simulink model "app_Main50msMgr"  (R2016b)
settings: Solver=FixedStepDiscrete  StartTime=0.0  StopTime=10.0  FixedStep=0.001  RelTol=1e-3  EnableMultiTasking=on
PreLoadFcn:
  | try
  |    tapas_types('load');
  | catch
  |   disp('TAPAS WARNING: Tapas Types could not be loaded ...');
  | end
  | 
  | try
  |   app_types('load');
  | catch
  |   currdir =pwd;
  |   try
  |     cd('..\app_types\');
  |     app_types('load');
  |     cd(currdir);
  |   catch
  |     try
  |        cd('..\..\app_types\');
  |        app_types('load');
  |        cd(currdir);
  |     catch
  |        cd(currdir);
  |        disp('TAPAS WARNING: Application Types could not be loaded ...');
  |     end
  |   end
  |   try
  |       clear currdir;
  |   catch
  |      %Do nothing
  |   end
  | end
settings Model: Creator=kmansour  LastModifiedBy=karim
settings DataIOCC: LimitDataPoints=on  SaveFormat=Array
settings OptimizationCC: LifeSpan=1
settings DebuggingCC: AllowSymbolicDim=off  SFUnexpectedBacktrackingDiag=warning  SFNoUnconditionalDefaultTransitionDiag=warning  SFExecutionAtInitializationDiag=none
settings HardwareCC: ProdBitPerPointer=32  ProdBitPerSizeT=32  ProdBitPerPtrDiffT=32  ProdLargestAtomicInteger=Long  ProdLargestAtomicFloat=Double  ProdWordSize=32  ProdHWDeviceType=Texas Instruments->TMS570 Cortex-R4
settings ModelReferenceCC: ModelReferenceNumInstancesAllowed=Single  PropagateSignalLabelsOutOfModel=off
settings RTWCC: SystemTargetFile=ert.tlc  GenCodeOnly=on  TemplateMakefile=ert_default_tmf  Description=Embedded Coder  GenerateReport=on  IncludeHyperlinkInReport=on  LaunchReport=on  GenerateTraceInfo=on  GenerateTraceReport=on  GenerateTraceReportSl=on  GenerateTraceReportSf=on  GenerateTraceReportEml=on
settings CodeAppCC: IgnoreCustomStorageClasses=off  MaxIdLength=63
settings ERTTargetCC: GenerateSampleERTMain=on  ERTSrcFileBannerTemplate=tapas_code_template.cgt  ERTHdrFileBannerTemplate=tapas_code_template.cgt  ERTDataSrcFileTemplate=tapas_code_template.cgt  ERTDataHdrFileTemplate=tapas_code_template.cgt  ERTCustomFileTemplate=example_file_process.tlc  ConvertIfToSwitch=off  SuppressUnreachableDefaultCases=off
settings ConfigComp: CovMetricSettings=dw  CovHtmlReporting=on  CovSaveCumulativeToWorkspaceVar=on  CovSaveSingleToWorkspaceVar=on  CovExternalEMLEnable=off

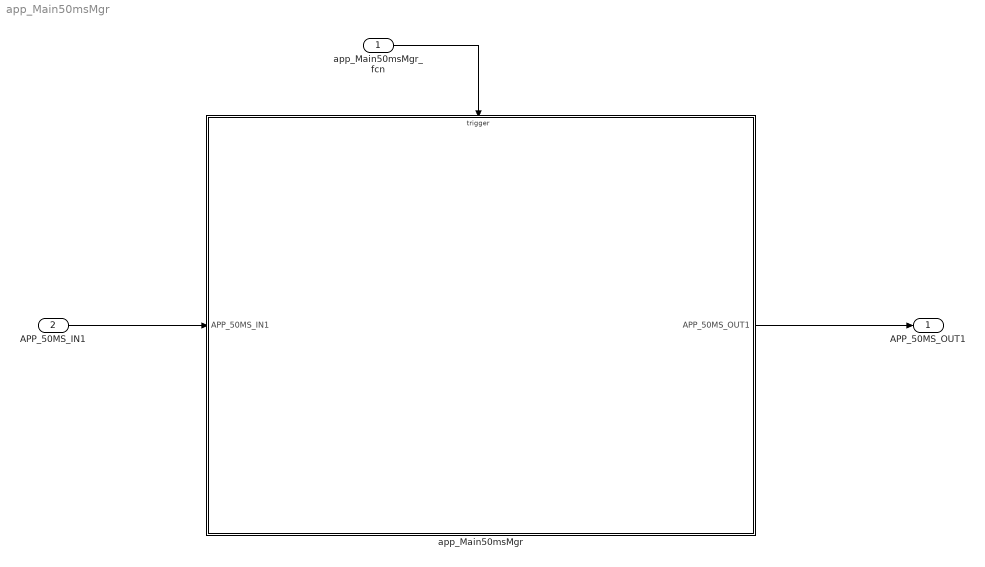
== system app_Main50msMgr ==
  app_Main50msMgr_fcn : Inport  SampleTime=50e-3  OutputFunctionCall=on
  APP_50MS_IN1 : Inport  Port=2
  app_Main50msMgr : Subsystem
  APP_50MS_OUT1 : Outport
  wires:
  app_Main50msMgr_fcn/1 -> app_Main50msMgr/Trigger
  APP_50MS_IN1/1 -> app_Main50msMgr/1(APP_50MS_IN1)
  app_Main50msMgr/1(APP_50MS_OUT1) -> APP_50MS_OUT1/1

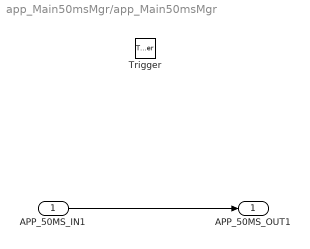
== system app_Main50msMgr/app_Main50msMgr ==
  APP_50MS_IN1 : Inport
  Trigger : TriggerPort  TriggerType=function-call  VariantControl=Variant  SampleTimeType=periodic  SampleTime=-1  PortDimensions=1
  APP_50MS_OUT1 : Outport
  wires:
  APP_50MS_IN1/1 -> APP_50MS_OUT1/1
